simulink model "TorqueDeratingandLimitingComponent"  (R2026a)
settings: Solver=FixedStepDiscrete
settings Model: DataDictionary=TractionEmotorSoftwareArchInterfaceData.sldd  Creator=dakaihu  LastModifiedBy=dakaihu

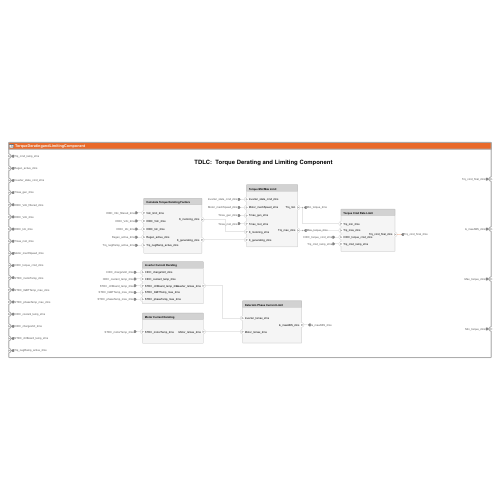
[thumbnail: Simulink's stored preview of the top-level diagram]
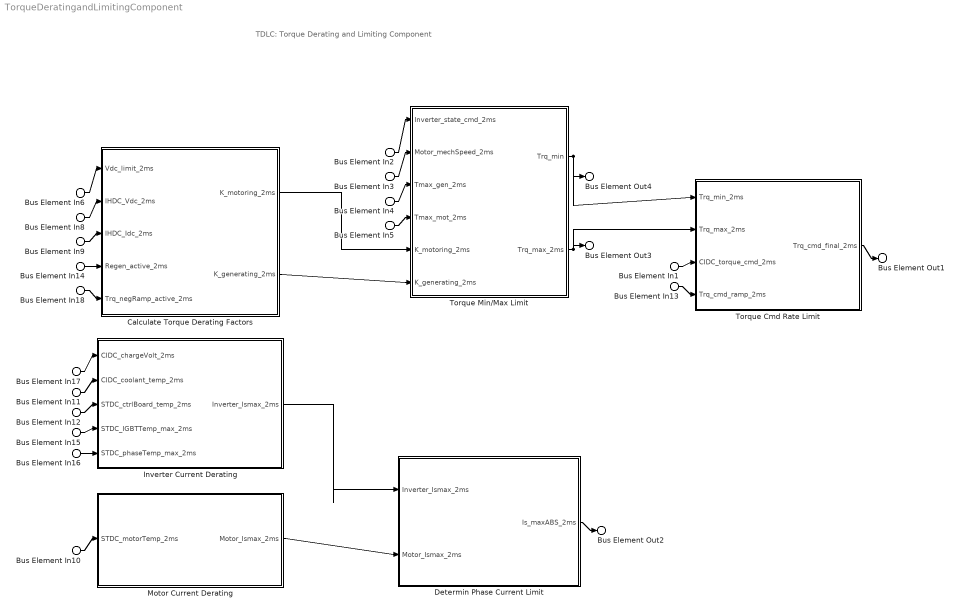
== system TorqueDeratingandLimitingComponent ==
  note: TDLC: Torque Derating and Limiting Component
  Bus Element In13 : Inport  PortName=Trq_cmd_ramp_2ms
  Bus Element In14 : Inport  Port=2  PortName=Regen_active_2ms
  Bus Element In2 : Inport  Port=3  PortName=Inverter_state_cmd_2ms
  Bus Element In4 : Inport  Port=4  PortName=Tmax_gen_2ms
  Bus Element In6 : Inport  Port=5  PortName=IHDC_Vdc_filtered_2ms
  Bus Element In8 : Inport  Port=6  PortName=IHDC_Vdc_2ms
  Bus Element In9 : Inport  Port=7  PortName=IHDC_Idc_2ms
  Bus Element In5 : Inport  Port=8  PortName=Tmax_mot_2ms
  Bus Element In3 : Inport  Port=9  PortName=Motor_mechSpeed_2ms
  Bus Element In1 : Inport  Port=10  PortName=CIDC_torque_cmd_2ms
  Bus Element In10 : Inport  Port=11  PortName=STDC_motorTemp_2ms
  Bus Element In15 : Inport  Port=12  PortName=STDC_IGBTTemp_max_2ms
  Bus Element In16 : Inport  Port=13  PortName=STDC_phaseTemp_max_2ms
  Bus Element In11 : Inport  Port=14  PortName=CIDC_coolant_temp_2ms
  Bus Element In17 : Inport  Port=15  PortName=CIDC_chargeVolt_2ms
  Bus Element In12 : Inport  Port=16  PortName=STDC_ctrlBoard_temp_2ms
  Bus Element In18 : Inport  Port=17  PortName=Trq_negRamp_active_2ms
  Calculate Torque Derating Factors : Subsystem
      settings: PortSchema="{\"entries\":[{\"content\":{\"headerSize\":26,\"margin\":15,\"minimumSpacing\":25,\"sides\":[{\"content\":{\"connectorIds\":[\"In1\",\"In2\",\"In3\",\"In4\",\"In5\"]},\"type\":\"ConnectorPlacement.EquallySpacedRectSide\",\"uuid\":\"fd31d295-2ee8-4010-a085-72a956fb88db\"},{\"content\":{\"connectorIds\":[\"Out1\",\"Out2\"],\"side\":\"RIGHT\"},\"type\":\"ConnectorPlacement.EquallySpacedRectSide\",\"uuid\":\"6e15e65a-8b2c-4657-b6d9-6871ed377dcc\"},{\"content\":{\"connectorIds\":[],\"side\":\"TOP\"},\"type\":\"ConnectorPlacement.EquallySpacedRectSide\",\"uuid\":\"e10f5a11-10a3-425e-91ff-fff14d159c09\"}]},\"type\":\"ConnectorPlacement.EquallySpacedConnector\",\"uuid\":\"062b7cf1-4df3-4671-ab85-e62a20780700\"}],\"packageUris\":[\"http://schema.mathworks.com/mf0/Connector/R2020b\"],\"version\":\"1.0\"}"
  Determin Phase Current Limit : Subsystem
      settings: PortSchema="{\"entries\":[{\"content\":{\"headerSize\":26,\"margin\":15,\"minimumSpacing\":25,\"sides\":[{\"content\":{\"connectorIds\":[\"In1\",\"In2\"]},\"type\":\"ConnectorPlacement.EquallySpacedRectSide\",\"uuid\":\"fd31d295-2ee8-4010-a085-72a956fb88db\"},{\"content\":{\"connectorIds\":[\"Out1\"],\"side\":\"RIGHT\"},\"type\":\"ConnectorPlacement.EquallySpacedRectSide\",\"uuid\":\"6e15e65a-8b2c-4657-b6d9-6871ed377dcc\"},{\"content\":{\"connectorIds\":[],\"side\":\"TOP\"},\"type\":\"ConnectorPlacement.EquallySpacedRectSide\",\"uuid\":\"e10f5a11-10a3-425e-91ff-fff14d159c09\"}]},\"type\":\"ConnectorPlacement.EquallySpacedConnector\",\"uuid\":\"062b7cf1-4df3-4671-ab85-e62a20780700\"}],\"packageUris\":[\"http://schema.mathworks.com/mf0/Connector/R2020b\"],\"version\":\"1.0\"}"
  Inverter Current Derating : Subsystem
      settings: PortSchema="{\"entries\":[{\"content\":{\"headerSize\":26,\"margin\":15,\"minimumSpacing\":25,\"sides\":[{\"content\":{\"connectorIds\":[\"In1\",\"In2\",\"In3\",\"In4\",\"In5\"]},\"type\":\"ConnectorPlacement.EquallySpacedRectSide\",\"uuid\":\"fd31d295-2ee8-4010-a085-72a956fb88db\"},{\"content\":{\"connectorIds\":[\"Out1\"],\"side\":\"RIGHT\"},\"type\":\"ConnectorPlacement.EquallySpacedRectSide\",\"uuid\":\"6e15e65a-8b2c-4657-b6d9-6871ed377dcc\"},{\"content\":{\"connectorIds\":[],\"side\":\"TOP\"},\"type\":\"ConnectorPlacement.EquallySpacedRectSide\",\"uuid\":\"e10f5a11-10a3-425e-91ff-fff14d159c09\"}]},\"type\":\"ConnectorPlacement.EquallySpacedConnector\",\"uuid\":\"062b7cf1-4df3-4671-ab85-e62a20780700\"}],\"packageUris\":[\"http://schema.mathworks.com/mf0/Connector/R2020b\"],\"version\":\"1.0\"}"
  Motor Current Derating : Subsystem
      settings: PortSchema="{\"entries\":[{\"content\":{\"headerSize\":26,\"margin\":15,\"minimumSpacing\":25,\"sides\":[{\"content\":{\"connectorIds\":[\"In1\"]},\"type\":\"ConnectorPlacement.EquallySpacedRectSide\",\"uuid\":\"fd31d295-2ee8-4010-a085-72a956fb88db\"},{\"content\":{\"connectorIds\":[\"Out1\"],\"side\":\"RIGHT\"},\"type\":\"ConnectorPlacement.EquallySpacedRectSide\",\"uuid\":\"6e15e65a-8b2c-4657-b6d9-6871ed377dcc\"},{\"content\":{\"connectorIds\":[],\"side\":\"TOP\"},\"type\":\"ConnectorPlacement.EquallySpacedRectSide\",\"uuid\":\"e10f5a11-10a3-425e-91ff-fff14d159c09\"}]},\"type\":\"ConnectorPlacement.EquallySpacedConnector\",\"uuid\":\"062b7cf1-4df3-4671-ab85-e62a20780700\"}],\"packageUris\":[\"http://schema.mathworks.com/mf0/Connector/R2020b\"],\"version\":\"1.0\"}"
  Torque Cmd Rate Limit : Subsystem
      settings: PortSchema="{\"entries\":[{\"content\":{\"headerSize\":26,\"margin\":15,\"minimumSpacing\":25,\"sides\":[{\"content\":{\"connectorIds\":[\"In1\",\"In2\",\"In3\",\"In4\"]},\"type\":\"ConnectorPlacement.EquallySpacedRectSide\",\"uuid\":\"fd31d295-2ee8-4010-a085-72a956fb88db\"},{\"content\":{\"connectorIds\":[\"Out1\"],\"side\":\"RIGHT\"},\"type\":\"ConnectorPlacement.EquallySpacedRectSide\",\"uuid\":\"6e15e65a-8b2c-4657-b6d9-6871ed377dcc\"},{\"content\":{\"connectorIds\":[],\"side\":\"TOP\"},\"type\":\"ConnectorPlacement.EquallySpacedRectSide\",\"uuid\":\"e10f5a11-10a3-425e-91ff-fff14d159c09\"}]},\"type\":\"ConnectorPlacement.EquallySpacedConnector\",\"uuid\":\"062b7cf1-4df3-4671-ab85-e62a20780700\"}],\"packageUris\":[\"http://schema.mathworks.com/mf0/Connector/R2020b\"],\"version\":\"1.0\"}"
  "Torque Min/Max Limit " : Subsystem
      settings: PortSchema="{\"entries\":[{\"content\":{\"headerSize\":26,\"margin\":15,\"minimumSpacing\":25,\"sides\":[{\"content\":{\"connectorIds\":[\"In6\",\"In1\",\"In2\",\"In3\",\"In4\",\"In5\"]},\"type\":\"ConnectorPlacement.EquallySpacedRectSide\",\"uuid\":\"fd31d295-2ee8-4010-a085-72a956fb88db\"},{\"content\":{\"connectorIds\":[\"Out2\",\"Out1\"],\"side\":\"RIGHT\"},\"type\":\"ConnectorPlacement.EquallySpacedRectSide\",\"uuid\":\"6e15e65a-8b2c-4657-b6d9-6871ed377dcc\"},{\"content\":{\"connectorIds\":[],\"side\":\"TOP\"},\"type\":\"ConnectorPlacement.EquallySpacedRectSide\",\"uuid\":\"e10f5a11-10a3-425e-91ff-fff14d159c09\"},{\"content\":{\"connectorIds\":[],\"side\":\"BOTTOM\"},\"type\":\"ConnectorPlacement.EquallySpacedRectSide\",\"uuid\":\"a64ea9c0-8db1-4f8e-8e7f-fc26b2bba70e\"}]},\"type\":\"ConnectorPlacement.EquallySpacedConnector\",\"uuid\":\"062b7cf1-4df3-4671-ab85-e62a20780700\"}],\"packageUris\":[\"http://schema.mathworks.com/mf0/Connector/R2020b\"],\"version\":\"1.0\"}"
  Bus Element Out1 : Outport  PortName=Trq_cmd_final_2ms
  Bus Element Out2 : Outport  Port=2  PortName=Is_maxABS_2ms
  Bus Element Out3 : Outport  Port=3  PortName=Max_torque_2ms
  Bus Element Out4 : Outport  Port=4  PortName=Min_torque_2ms
  wires:
  Bus Element In1/1 -> Torque Cmd Rate Limit/3(CIDC_torque_cmd_2ms)
  "Torque Min/Max Limit "/1(Trq_max_2ms) -> Torque Cmd Rate Limit/2(Trq_max_2ms), Bus Element Out3/1
  "Torque Min/Max Limit "/2(Trq_min) -> Torque Cmd Rate Limit/1(Trq_min_2ms), Bus Element Out4/1
  Calculate Torque Derating Factors/1(K_motoring_2ms) -> "Torque Min/Max Limit "/4(K_motoring_2ms)
  Calculate Torque Derating Factors/2(K_generating_2ms) -> "Torque Min/Max Limit "/5(K_generating_2ms)
  Bus Element In2/1 -> "Torque Min/Max Limit "/6(Inverter_state_cmd_2ms)
  Bus Element In3/1 -> "Torque Min/Max Limit "/1(Motor_mechSpeed_2ms)
  Bus Element In4/1 -> "Torque Min/Max Limit "/2(Tmax_gen_2ms)
  Bus Element In5/1 -> "Torque Min/Max Limit "/3(Tmax_mot_2ms)
  Bus Element In6/1 -> Calculate Torque Derating Factors/1(Vdc_limit_2ms)
  Bus Element In8/1 -> Calculate Torque Derating Factors/2(IHDC_Vdc_2ms)
  Bus Element In9/1 -> Calculate Torque Derating Factors/3(IHDC_Idc_2ms)
  Motor Current Derating/1(Motor_Ismax_2ms) -> Determin Phase Current Limit/2(Motor_Ismax_2ms)
  Inverter Current Derating/1(Inverter_Ismax_2ms) -> Determin Phase Current Limit/1(Inverter_Ismax_2ms)
  Bus Element In10/1 -> Motor Current Derating/1(STDC_motorTemp_2ms)
  Bus Element In11/1 -> Inverter Current Derating/2(CIDC_coolant_temp_2ms)
  Bus Element In12/1 -> Inverter Current Derating/3(STDC_ctrlBoard_temp_2ms)
  Bus Element In13/1 -> Torque Cmd Rate Limit/4(Trq_cmd_ramp_2ms)
  Torque Cmd Rate Limit/1(Trq_cmd_final_2ms) -> Bus Element Out1/1
  Determin Phase Current Limit/1(Is_maxABS_2ms) -> Bus Element Out2/1
  Bus Element In14/1 -> Calculate Torque Derating Factors/4(Regen_active_2ms)
  Bus Element In15/1 -> Inverter Current Derating/4(STDC_IGBTTemp_max_2ms)
  Bus Element In16/1 -> Inverter Current Derating/5(STDC_phaseTemp_max_2ms)
  Bus Element In17/1 -> Inverter Current Derating/1(CIDC_chargeVolt_2ms)
  Bus Element In18/1 -> Calculate Torque Derating Factors/5(Trq_negRamp_active_2ms)

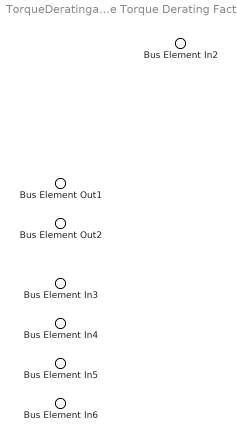
== system TorqueDeratingandLimitingComponent/Calculate Torque Derating Factors ==
  Bus Element In2 : Inport  PortName=Vdc_limit_2ms
  Bus Element In3 : Inport  Port=2  PortName=IHDC_Vdc_2ms
  Bus Element In4 : Inport  Port=3  PortName=IHDC_Idc_2ms
  Bus Element In5 : Inport  Port=4  PortName=Regen_active_2ms
  Bus Element In6 : Inport  Port=5  PortName=Trq_negRamp_active_2ms
  Bus Element Out1 : Outport  PortName=K_motoring_2ms
  Bus Element Out2 : Outport  Port=2  PortName=K_generating_2ms

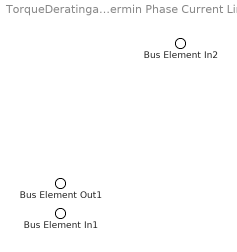
== system TorqueDeratingandLimitingComponent/Determin Phase Current Limit ==
  Bus Element In2 : Inport  PortName=Inverter_Ismax_2ms
  Bus Element In1 : Inport  Port=2  PortName=Motor_Ismax_2ms
  Bus Element Out1 : Outport  PortName=Is_maxABS_2ms

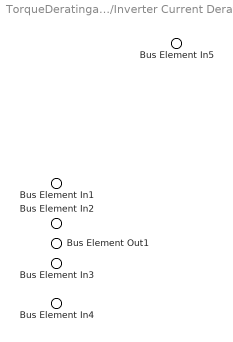
== system TorqueDeratingandLimitingComponent/Inverter Current Derating ==
  Bus Element In5 : Inport  PortName=CIDC_chargeVolt_2ms
  Bus Element In1 : Inport  Port=2  PortName=CIDC_coolant_temp_2ms
  Bus Element In2 : Inport  Port=3  PortName=STDC_ctrlBoard_temp_2ms
  Bus Element In3 : Inport  Port=4  PortName=STDC_IGBTTemp_max_2ms
  Bus Element In4 : Inport  Port=5  PortName=STDC_phaseTemp_max_2ms
  Bus Element Out1 : Outport  PortName=Inverter_Ismax_2ms

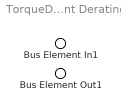
== system TorqueDeratingandLimitingComponent/Motor Current Derating ==
  Bus Element In1 : Inport  PortName=STDC_motorTemp_2ms
  Bus Element Out1 : Outport  PortName=Motor_Ismax_2ms

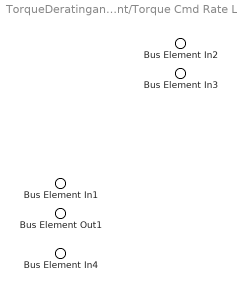
== system TorqueDeratingandLimitingComponent/Torque Cmd Rate Limit ==
  Bus Element In3 : Inport  PortName=Trq_min_2ms
  Bus Element In2 : Inport  Port=2  PortName=Trq_max_2ms
  Bus Element In1 : Inport  Port=3  PortName=CIDC_torque_cmd_2ms
  Bus Element In4 : Inport  Port=4  PortName=Trq_cmd_ramp_2ms
  Bus Element Out1 : Outport  PortName=Trq_cmd_final_2ms

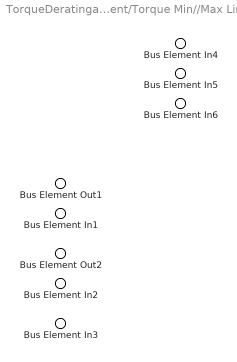
== system TorqueDeratingandLimitingComponent/Torque Min//Max Limit  ==
  Bus Element In4 : Inport  PortName=Motor_mechSpeed_2ms
  Bus Element In5 : Inport  Port=2  PortName=Tmax_gen_2ms
  Bus Element In6 : Inport  Port=3  PortName=Tmax_mot_2ms
  Bus Element In1 : Inport  Port=4  PortName=K_motoring_2ms
  Bus Element In2 : Inport  Port=5  PortName=K_generating_2ms
  Bus Element In3 : Inport  Port=6  PortName=Inverter_state_cmd_2ms
  Bus Element Out1 : Outport  PortName=Trq_max_2ms
  Bus Element Out2 : Outport  Port=2  PortName=Trq_min
